simulink model "furuta_ppo"  (R2015b)
settings: Solver=FixedStepDiscrete  StartTime=0.0  StopTime=inf  FixedStep=0.002  RelTol=1e-3
values from neighbouring files (symbols this model uses):
  A_aug = [A Bz; zeros(2,6)]    [Furuta_Pendulum_bring_down.m]    (also in Furuta_Pendulum_up_pos.m)
  B_aug = [B ;0;0]    [Furuta_Pendulum_bring_down.m]    (also in Furuta_Pendulum_up_pos.m)
  C_aug = [C zeros(2,2)]    [Furuta_Pendulum_bring_down.m]    (also in Furuta_Pendulum_up_pos.m)
  I_max = 0.5    [Furuta_Pendulum_bring_down.m]    (also in Furuta_Pendulum_up_pos.m = 0.8)
  Km = 7.86e-3    (= 0.00786)    [Furuta_Pendulum_bring_down.m]    (also in Furuta_Pendulum_up_pos.m)
  L_aug = real (L1+L2+L3)    [Furuta_Pendulum_bring_down.m]    (also in Furuta_Pendulum_up_pos.m)
  N = 70    [Furuta_Pendulum_bring_down.m]    (also in Furuta_Pendulum_up_pos.m)
  nu = 0.9    [Furuta_Pendulum_bring_down.m]    (also in Furuta_Pendulum_up_pos.m)
  Qz = - inv(Cr1*inv(Ar-Br*r')*Br)*Cr1*inv(Ar-Br*r')*Bzr    [Furuta_Pendulum_bring_down.m]    (also in Furuta_Pendulum_up_pos.m = inv(Cr1*inv(Ar-Br*r')*Br)*Cr1*inv(Ar-Br*r')*Bzr)
  R = 2.75    [Furuta_Pendulum_bring_down.m]    (also in Furuta_Pendulum_up_pos.m)
  Tr = [Su(end,:) ; Su(end,:)*A; Su(end,:)*A^2;Su(end,:)*A^3]    [Furuta_Pendulum_bring_down.m]    (also in Furuta_Pendulum_up_pos.m)
  V_max = 5    [Furuta_Pendulum_bring_down.m]    (also in Furuta_Pendulum_up_pos.m = 8)
undefined symbols (not defined in the file or in its folder): HIL, qc_get_step_size
libraries: quarc_library x5, simulink x3
settings Model: ExtModeTrigDuration=10000  Creator=sgillen  LastModifiedBy=sgillen
settings SolverCC: PositivePriorityOrder=on
settings RTWCC: SystemTargetFile=quarc_win64.tlc  TemplateMakefile=quarc_default_tmf  Description=QUARC Win64 Target
settings STFCustomTargetCC: GeneratePreprocessorConditionals=Use local settings  CPPClassGenCompliant=off
settings GRTTargetCC: ParMdlRefBuildCompliant=off  CompOptLevelCompliant=off  CombineOutputUpdateFcns=off  MatFileLogging=off  CPPClassGenCompliant=off  GRTInterface=on  UseToolchainInfoCompliant=off  ExtMode=on  ExtModeMexFile=quarc_comm

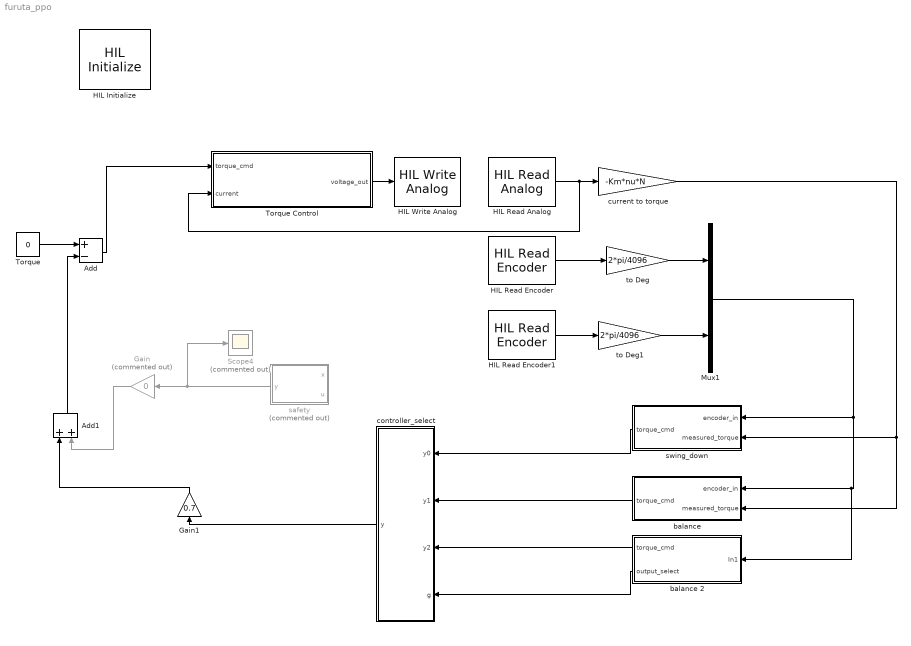
== system furuta_ppo ==
  Add : Sum  Inputs=+-
  Add1 : Sum
  Gain : Gain  Commented=on  Gain=0
  Gain1 : Gain  Gain=0.7
  HIL Initialize : quarc_library/Data Acquisition/Generic/Configuration/HIL Initialize  object_name=HIL-1  board_type=q4  board_number=0  board_options=""  exclusive=off  active=on  hardware_clocks=[0:1]  clock_modes=[0 0]  initial_clock_frequencies=[]  set_clock_params_at_start=on  set_clock_params_at_switch_in=off  set_clock_frequencies_at_start=off  set_clock_frequencies_at_switch_in=off  analog_input_channels=[0:3]  analog_input_configurations=[]  analog_input_maximums=10  analog_input_minimums=-10  set_analog_input_params_at_start=off  set_analog_input_params_at_switch_in=off  analog_output_channels=[0:3]  analog_output_maximums=[10]  analog_output_minimums=[-10]  initial_analog_outputs=[0]  final_analog_outputs=[0]  watchdog_analog_outputs=0  set_analog_output_params_at_start=on  set_analog_output_params_at_switch_in=off  set_analog_outputs_at_start=on  set_analog_outputs_at_switch_in=off  set_analog_outputs_at_terminate=on  set_analog_outputs_at_switch_out=off  set_analog_outputs_on_watchdog=off  digital_input_channels=[]  digital_output_channels=[]  digital_output_configuration=[]  initial_digital_outputs=[1]  final_digital_outputs=[1]  watchdog_digital_outputs=[2]  set_digital_output_params_at_start=off  set_digital_output_params_at_switch_in=off  set_digital_outputs_at_start=on  set_digital_outputs_at_switch_in=off  set_digital_outputs_at_terminate=on  set_digital_outputs_at_switch_out=off  set_digital_outputs_on_watchdog=off  encoder_channels=[0:3]  quadrature=[4]  encoder_filter_frequency=(1/60e-9)/1  initial_encoder_counts=[0]  set_encoder_params_at_start=on  set_encoder_params_at_switch_in=off  set_encoder_counts_at_start=on  set_encoder_counts_at_switch_in=off  pwm_channels=[]  pwm_modes=[0]  pwm_frequency=(1/60e-9)/1024  pwm_configuration=[]  pwm_alignment=[]  pwm_polarity=[]  pwm_leading_deadband=[]  pwm_trailing_deadband=[]  initial_pwm_outputs=[0]  final_pwm_outputs=[0]  watchdog_pwm_outputs=[]  set_pwm_params_at_start=on  set_pwm_params_at_switch_in=off  set_pwm_outputs_at_start=on  set_pwm_outputs_at_switch_in=off  set_pwm_outputs_at_terminate=on  set_pwm_outputs_at_switch_out=off  set_pwm_outputs_on_watchdog=off  other_output_channels=[]  initial_other_outputs=[]  final_other_outputs=[]  watchdog_other_outputs=[]  set_other_outputs_at_start=off  set_other_outputs_at_switch_in=off  set_other_outputs_at_terminate=off  set_other_outputs_at_switch_out=off  set_other_outputs_on_watchdog=off
  HIL Read Analog : quarc_library/Data Acquisition/Generic/Immediate I//O/HIL Read Analog  object_name=HIL-1  channels=1  sample_time=qc_get_step_size  active=on  vector_output=off
  HIL Read Encoder : quarc_library/Data Acquisition/Generic/Immediate I//O/HIL Read Encoder  object_name=HIL-1  channels=0  sample_time=qc_get_step_size  active=on  vector_output=off  data_type_mode=Inherit via back propagation  data_type=double
  HIL Read Encoder1 : quarc_library/Data Acquisition/Generic/Immediate I//O/HIL Read Encoder  object_name=HIL-1  channels=1  sample_time=qc_get_step_size  active=on  vector_output=off  data_type_mode=Inherit via back propagation  data_type=double
  HIL Write Analog : quarc_library/Data Acquisition/Generic/Immediate I//O/HIL Write Analog  object_name=HIL-1  channels=0  sample_time=-1  active=off  vector_input=off
  Mux1 : Mux  Inputs=2
  Scope4 : Scope  Commented=on
  Torque : Constant  Value=0
  Torque Control : Subsystem
  "balance " : Subsystem
  balance 2 : Subsystem
  "controller_select " : MATLAB Function  TreatAsAtomicUnit=on
  current to torque : Gain  Gain=-Km*nu*N
  safety : MATLAB Function  Commented=on  TreatAsAtomicUnit=on
  swing_down : Subsystem
  to Deg : Gain  Gain=2*pi/4096
  to Deg1 : Gain  Gain=2*pi/4096
  wires:
  HIL Read Encoder/1 -> to Deg/1
  HIL Read Encoder1/1 -> to Deg1/1
  to Deg1/1 -> Mux1/2
  to Deg/1 -> Mux1/1
  Torque/1 -> Add/1
  Add/1 -> Torque Control/1("torque_cmd ")
  safety/1(y) -> Gain/1, Scope4/1
  Gain1/1 -> Add1/1
  Add1/1 -> Add/2
  Gain/1 -> Add1/2
  Torque Control/1("voltage_out ") -> HIL Write Analog/1
  HIL Read Analog/1 -> Torque Control/2(current), current to torque/1
  current to torque/1 -> swing_down/2(measured_torque), "balance "/2(measured_torque)
  Mux1/1 -> swing_down/1("encoder_in "), balance 2/1(In1), "balance "/1("encoder_in ")
  balance 2/2("output_select ") -> "controller_select "/4(g)
  "balance "/1("torque_cmd ") -> "controller_select "/2(y1)
  swing_down/1("torque_cmd ") -> "controller_select "/1(y0)
  balance 2/1(torque_cmd) -> "controller_select "/3(y2)
  "controller_select "/1(y) -> Gain1/1

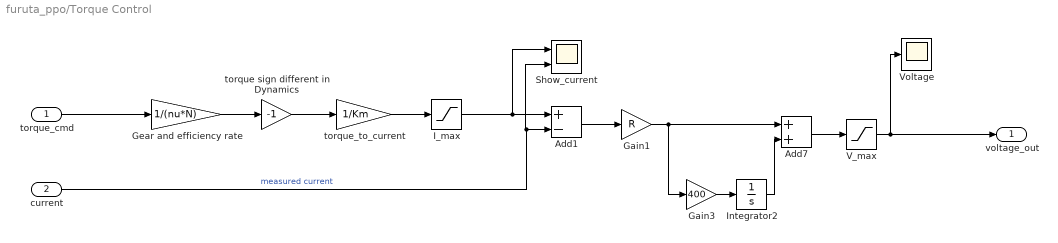
== system furuta_ppo/Torque Control ==
  "torque_cmd " : Inport
  current : Inport  Port=2
  Add1 : Sum  Inputs=+-
  Add7 : Sum
  Gain1 : Gain  Gain=R
  Gain3 : Gain  Gain=400
  Gear and efficiency rate : Gain  Gain=1/(nu*N)
  I_max : Saturate  UpperLimit=I_max  LowerLimit=-I_max
  Integrator2 : Integrator
  Show_current : Scope  NumInputPorts=2
  V_max : Saturate  UpperLimit=V_max  LowerLimit=-V_max
  Voltage : Scope
  torque sign different in Dynamics : Gain  Gain=-1
  torque_to_current : Gain  Gain=1/Km
  "voltage_out " : Outport
  wires:
  Gear and efficiency rate/1 -> torque sign different in Dynamics/1
  current/1 -> Add1/2, Show_current/2  "measured current"
  Add1/1 -> Gain1/1
  torque sign different in Dynamics/1 -> torque_to_current/1
  Add7/1 -> V_max/1
  I_max/1 -> Show_current/1, Add1/1
  Gain3/1 -> Integrator2/1
  Gain1/1 -> Add7/1, Gain3/1
  V_max/1 -> "voltage_out "/1, Voltage/1
  Integrator2/1 -> Add7/2
  torque_to_current/1 -> I_max/1
  "torque_cmd "/1 -> Gear and efficiency rate/1

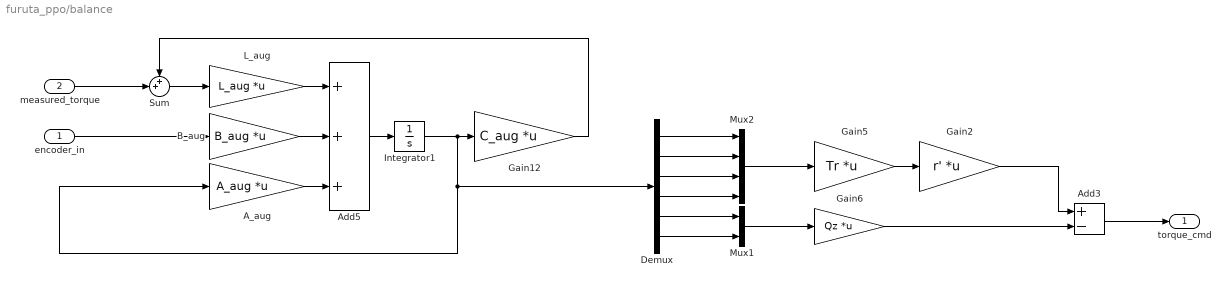
== system furuta_ppo/balance  ==
  "encoder_in " : Inport
  measured_torque : Inport  Port=2
  A_aug : Gain  Gain=A_aug  Multiplication=Matrix(K*u) (u vector)
  Add3 : Sum  Inputs=+-
  Add5 : Sum  Inputs=+++
  B_aug : Gain  Gain=B_aug  Multiplication=Matrix(K*u) (u vector)
  Demux : Demux  Outputs=6
  Gain12 : Gain  Gain=C_aug  Multiplication=Matrix(K*u) (u vector)
  Gain2 : Gain  Gain=r'  Multiplication=Matrix(K*u) (u vector)
  Gain5 : Gain  Gain=Tr  Multiplication=Matrix(K*u) (u vector)
  Gain6 : Gain  Gain=Qz  Multiplication=Matrix(K*u) (u vector)
  Integrator1 : Integrator
  "L_aug " : Gain  Gain=L_aug  Multiplication=Matrix(K*u) (u vector)
  Mux1 : Mux  Inputs=2
  Mux2 : Mux
  Sum : Sum  Inputs=++|
  "torque_cmd " : Outport
  wires:
  Integrator1/1 -> Gain12/1, A_aug/1, Demux/1
  Add5/1 -> Integrator1/1
  Gain12/1 -> Sum/1
  A_aug/1 -> Add5/3
  B_aug/1 -> Add5/2
  "L_aug "/1 -> Add5/1
  "encoder_in "/1 -> B_aug/1
  measured_torque/1 -> Sum/2
  Sum/1 -> "L_aug "/1
  Mux2/1 -> Gain5/1
  Gain5/1 -> Gain2/1
  Gain2/1 -> Add3/1
  Gain6/1 -> Add3/2
  Mux1/1 -> Gain6/1
  Add3/1 -> "torque_cmd "/1
  Demux/1 -> Mux2/1
  Demux/2 -> Mux2/2
  Demux/3 -> Mux2/3
  Demux/4 -> Mux2/4
  Demux/5 -> Mux1/1
  Demux/6 -> Mux1/2

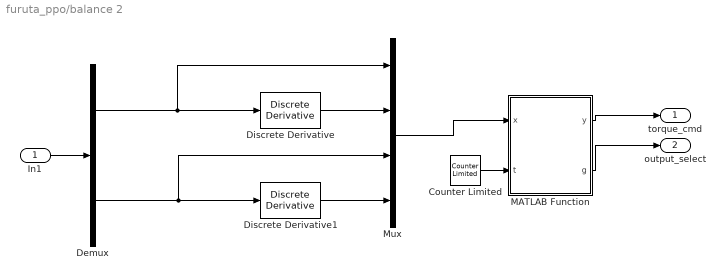
== system furuta_ppo/balance 2 ==
  In1 : Inport
  Counter Limited : simulink/Sources/Counter Limited  uplimit=.2/qc_get_step_size;  tsamp=-1
  Demux : Demux  Outputs=2
  Discrete Derivative : simulink/Discrete/Discrete Derivative  gainval=1.0  ICPrevScaledInput=0.0  InputProcessing=Inherited  OutMin=[]  OutMax=[]  OutDataType=fixdt(1, 16)  OutScaling=2^-10  DoSatur=off
  Discrete Derivative1 : simulink/Discrete/Discrete Derivative  gainval=1.0  ICPrevScaledInput=0.0  InputProcessing=Inherited  OutMin=[]  OutMax=[]  OutDataType=fixdt(1, 16)  OutScaling=2^-10  DoSatur=off
  MATLAB Function : MATLAB Function  TreatAsAtomicUnit=on
  Mux : Mux
  torque_cmd : Outport
  "output_select " : Outport  Port=2
  wires:
  Demux/2 -> Mux/3, Discrete Derivative1/1
  Discrete Derivative/1 -> Mux/2
  Discrete Derivative1/1 -> Mux/4
  Mux/1 -> MATLAB Function/1(x)
  Counter Limited/1 -> MATLAB Function/2(t)
  MATLAB Function/1(y) -> torque_cmd/1
  MATLAB Function/2(g) -> "output_select "/1
  Demux/1 -> Mux/1, Discrete Derivative/1
  In1/1 -> Demux/1

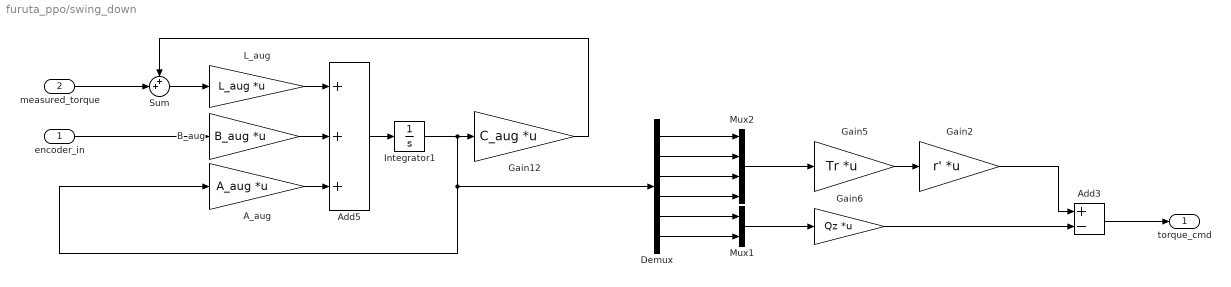
== system furuta_ppo/swing_down ==
  "encoder_in " : Inport
  measured_torque : Inport  Port=2
  A_aug : Gain  Gain=A_aug  Multiplication=Matrix(K*u) (u vector)
  Add3 : Sum  Inputs=+-
  Add5 : Sum  Inputs=+++
  B_aug : Gain  Gain=B_aug  Multiplication=Matrix(K*u) (u vector)
  Demux : Demux  Outputs=6
  Gain12 : Gain  Gain=C_aug  Multiplication=Matrix(K*u) (u vector)
  Gain2 : Gain  Gain=r'  Multiplication=Matrix(K*u) (u vector)
  Gain5 : Gain  Gain=Tr  Multiplication=Matrix(K*u) (u vector)
  Gain6 : Gain  Gain=Qz  Multiplication=Matrix(K*u) (u vector)
  Integrator1 : Integrator
  "L_aug " : Gain  Gain=L_aug  Multiplication=Matrix(K*u) (u vector)
  Mux1 : Mux  Inputs=2
  Mux2 : Mux
  Sum : Sum  Inputs=++|
  "torque_cmd " : Outport
  wires:
  Integrator1/1 -> Gain12/1, A_aug/1, Demux/1
  Add5/1 -> Integrator1/1
  Gain12/1 -> Sum/1
  A_aug/1 -> Add5/3
  B_aug/1 -> Add5/2
  "L_aug "/1 -> Add5/1
  "encoder_in "/1 -> B_aug/1
  measured_torque/1 -> Sum/2
  Sum/1 -> "L_aug "/1
  Mux2/1 -> Gain5/1
  Gain5/1 -> Gain2/1
  Gain2/1 -> Add3/1
  Gain6/1 -> Add3/2
  Mux1/1 -> Gain6/1
  Add3/1 -> "torque_cmd "/1
  Demux/1 -> Mux2/1
  Demux/2 -> Mux2/2
  Demux/3 -> Mux2/3
  Demux/4 -> Mux2/4
  Demux/5 -> Mux1/1
  Demux/6 -> Mux1/2

== matlab function furuta_ppo/safety ==
  data: x input; u input; y output
function y = fcn(x,u)
%% Parameter / Saturration
velocity_max = 1;
pos_max = 0.5 ; %pi/5
saturation = 0 ; % torque max is 0.2476 Nm

%%
phi1 = x(1);
phi2 = x(2);
vel1 = x(3); % velocity motor
vel2 = x(4); % velocity pendulum

 
if abs(phi1)>= pos_max % abs(vel1) >= velocity_max && 
    y = saturation;
    y = 0.2*sign(phi1)
else
    y = u;
end

== matlab function furuta_ppo/balance 2/MATLAB Function ==
  settings: updateMethod=DISCRETE  sampleTime=qc_get_step_size
  data: x input; y output; t input; g output
function [y,g]= ffnn(x, t) % might make these global in a second...
%fully connected network
persistent w, persistent b
persistent obs_mat, persistent act_mat
persistent y_last, persistent t_persistent
persistent weight_names, persistent bias_names

fd = fopen('test.dat');
qc_get_step_size = 1e-3;
dt = 2;
frame_skip = dt/qc_get_step_size;

std = .1;
hsize = 24;
ep_length = 100;

num_weights = 2*(hsize^2) + hsize*5 + hsize*3 + 1

%% saturation, safety 
velocity_max = 1;
pos_max = 0.5 ; %pi/5
saturation = 0 ; % torque max is 0.2476 Nm
phi1 = x(1); % pos motor
vel1 = x(3); % velocity motor

%%
% init persistent state
% -------------------------------------
if isempty(w) || isempty(b) || isempty(obs_mat) || isempty(act_mat) || isempty(t_persistent) || isempty(y_last)  || isempty(weight_names) || isempty(bias_names)
    w = {rand(4,hsize)/sqrt(num_weights), rand(hsize,hsize)/sqrt(num_weights), rand(hsize, hsize)/sqrt(num_weights), rand(hsize,1)/sqrt(num_weights)};
    b = {rand(hsize,1)/sqrt(num_weights), rand(hsize,1)/sqrt(num_weights), rand(hsize,1)/sqrt(num_weights), rand(1,1)/sqrt(num_weights)};
    obs_mat = zeros(ep_length,4);
    act_mat = zeros(ep_length,1);
    y_last = 0;
    t_persistent = 0;   
    weight_names = {'wght0.dat', 'wght1.dat', 'wght2.dat', 'wght3.dat'};
    bias_names   = {'bias0.dat', 'bias1.dat', 'bias2.dat', 'bias3.dat'};

end

obs_mat(t+1,:) = x

if t == 1 && t_persistent~=t

    %% load the weights
    
    % guess external functions are out too... I hate my life
    f = fopen(weight_names{1}, 'r'); w{1} = fread(f, [4, hsize], 'float'); fclose(f);
    f = fopen(weight_names{2}, 'r'); w{1} = fread(f, [hsize, hsize], 'float'); fclose(f);
    f = fopen(weight_names{3}, 'r'); w{1} = fread(f, [hsize, hsize], 'float'); fclose(f);
    f = fopen(weight_names{4}, 'r'); w{1} = fread(f, [hsize, 1], 'float'); fclose(f);

    f = fopen(bias_names{1}, 'r'); b{1} = fread(f, [1, hsize], 'float'); fclose(f);
    f = fopen(bias_names{2}, 'r'); b{1} = fread(f, [1, hsize], 'float'); fclose(f);
    f = fopen(bias_names{3}, 'r'); b{1} = fread(f, [1, hsize], 'float'); fclose(f);
    f = fopen(bias_names{4}, 'r'); b{1} = fread(f, [1,1], 'float'); fclose(f);

   
    %w{1} = read_weights(weight_names{1},4,hsize);
    %w{2} = read_weights(weight_names{2},hsize,hsize);
    %w{3} = read_weights(weight_names{3},hsize,hsize);
    %w{4} = read_weights(weight_names{4},hsize,1);

    %b{1} = read_weights(bias_names{1}, hsize, 1);
    %b{2} = read_weights(bias_names{2}, hsize, hsize);
    %b{3} = read_weights(bias_names{3}, hsize, hsize);
    %b{4} = read_weights(bias_names{4}, 1,1);
    
    
    % do nn calculation
    % -------------------------------------

    size_w = size(w);
    num_layers = size_w(2);

    
    % code gen doesn't support indexing cell arrays with variables...
    % xi = x';
    % for i = 1:num_layers-1
    %     xi = w{i}'*xi + b{i};
    %     xi = tanh(xi);
    % end

    %fine
    x1 = tanh(w{1}'*x + b{1})
    x2 = tanh(w{2}'*x1 + b{2})
    x3 = tanh(w{3}'*x2 + b{3})
    mean = w{end}'*x3;
    %mean = w{end}'*x3 + b{end};
    y = (randn*std + mean)
    y_last = y;
    
    if abs(phi1)>= pos_max % abs(vel1) >= velocity_max && 
        y = saturation;
        y = 0.2*sign(phi1)
        y_last = y
    end    

else
    y = y_last;
end

t_persistent = double(t);

% record obs and action (and logprob and state?)
% -------------------------------------
obs_mat(t+1,:) = x
act_mat(t+1,:) = y

end

function A= read_weights(file_name, dim1,dim2)
    f = fopen(file_name, 'r')
    A = fread(f, [dim1, dim2], 'double')
    fclose(f)
end

function write_weights(file_name, A)
    f = fopen(file_name, 'w');
    fwrite(f,A,'float64');
    fclose(f)
end

== matlab function furuta_ppo/controller_select  ==
  data: y0 input; y1 input; y2 input; y output; g input
function y = select_controller(y0,y1,y2,g)
    switch g
        case 0
            y = y0
        case 1
            y = y1
        case 2
            y = y2
    end 
end
